simulink model "PD_trajectory"  (R2020b)
settings: Solver=VariableStepAuto  StartTime=0.0  StopTime=10  RelTol=1e-3
libraries: pid_lib x6
(part 1 of 3)
settings Model: Creator=Asus  LastModifiedBy=Asus

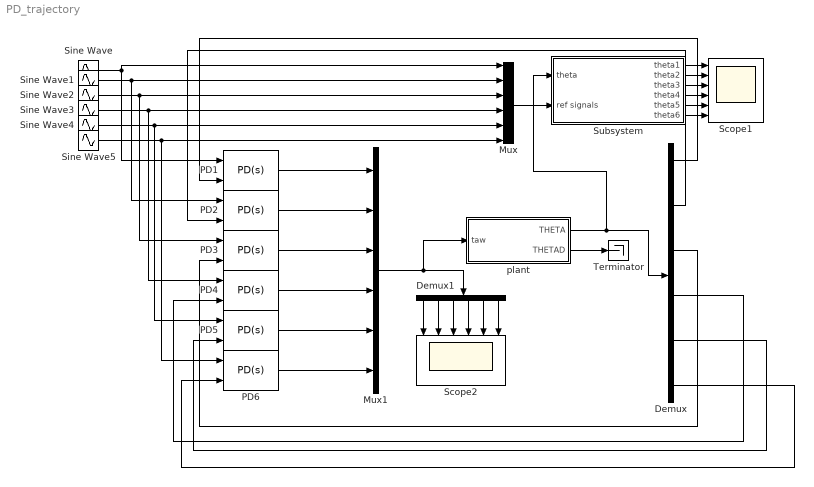
== system PD_trajectory ==
  Demux : Demux  Outputs=6
  Demux1 : Demux  Outputs=6
  Mux : Mux  Inputs=6
  Mux1 : Mux  Inputs=6
  PD1 : pid_lib/PID Controller (2DOF)  Controller=PD  Form=Parallel  TimeDomain=Continuous-time  UseExternalTs=off  SampleTime=-1  IntegratorMethod=Forward Euler  FilterMethod=Forward Euler  ControllerParametersSource=internal  P=343.666716329058  I=1  D=96720102.4595085  UseFilter=on  N=52762.3209030564  b=0.99828255964544  c=1.00028516180001  TunerSelectOption=Transfer Function Based (PID Tuner App)  InitialConditionSource=internal  InitialConditionForIntegrator=0  InitialConditionForFilter=0  DifferentiatorICPrevScaledInput=0  ExternalReset=none  TrackingMode=off  Kt=1  LimitOutput=off  SatLimitsSource=internal  UpperSaturationLimit=inf  LowerSaturationLimit=-inf  LinearizeAsGain=on  AntiWindupMode=none  Kb=1  POutMin=[]  POutMax=[]  IOutMin=[]  IOutMax=[]  DOutMin=[]  DOutMax=[]  NOutMin=[]  NOutMax=[]  bOutMin=[]  bOutMax=[]  cOutMin=[]  cOutMax=[]  SumOutMin=[]  SumOutMax=[]  SaturationOutMin=[]  SaturationOutMax=[]  PParamMin=[]  PParamMax=[]  IParamMin=[]  IParamMax=[]  DParamMin=[]  DParamMax=[]  NParamMin=[]  NParamMax=[]  bParamMin=[]  bParamMax=[]  cParamMin=[]  cParamMax=[]  KbParamMin=[]  KbParamMax=[]  KtParamMin=[]  KtParamMax=[]  KbOutMin=[]  KbOutMax=[]  KtOutMin=[]  KtOutMax=[]  IntegratorOutMin=[]  IntegratorOutMax=[]  FilterOutMin=[]  FilterOutMax=[]  SumI1OutMin=[]  SumI1OutMax=[]  SumI2OutMin=[]  SumI2OutMax=[]  SumI3OutMin=[]  SumI3OutMax=[]  SumI4OutMin=[]  SumI4OutMax=[]  SumDOutMin=[]  SumDOutMax=[]  Sum1OutMin=[]  Sum1OutMax=[]  Sum2OutMin=[]  Sum2OutMax=[]  Sum3OutMin=[]  Sum3OutMax=[]  DifferentiatorOutMin=[]  DifferentiatorOutMax=[]  FilterDiffOutCoefMin=[]  FilterDiffOutCoefMax=[]  ReciprocalOutMin=[]  ReciprocalOutMax=[]  SumDenOutMin=[]  SumDenOutMax=[]  SumNumOutMin=[]  SumNumOutMax=[]  DivideOutMin=[]  DivideOutMax=[]  UdiffTsProdOutMin=[]  UdiffTsProdOutMax=[]  NTsProdOutMin=[]  NTsProdOutMax=[]  UintegralTsProdOutMin=[]  UintegralTsProdOutMax=[]  UngainTsProdOutMin=[]  UngainTsProdOutMax=[]  IntegratorContinuousStateAttributes=''  IntegratorStateMustResolveToSignalObject=off  IntegratorRTWStateStorageClass=Auto  FilterContinuousStateAttributes=''  FilterStateMustResolveToSignalObject=off  FilterRTWStateStorageClass=Auto  ParallelPVariant=InternalParameters  IdealPVariant=Disabled  IVariant=Disabled  DVariant=InternalParameters  bVariant=InternalParameters  cVariant=InternalParameters  IntegratorVariant=Disabled  SatVariant=Disabled  AWVariant=Disabled  PCopyVariant=Disabled  TRVariant=Disabled  FdbkBlocksVariant=Forward  IdealPFdbkVariant=Disabled  SatFdbkVariant=Disabled  DerivativeFilterVariant=ContFilter  NVariant=InternalParameters  NCopyVariant=Disabled  FilterICVariant=InternalICsFilter  IntegratorICVariant=Disabled  ExternalResetVariant=Disabled  TRSumVariant=Passthrough  SumFdbkVariant=Disabled  SumVariant=Sum_PD  TsampFilterVariant=InternalTs  TsampNgainVariant=Passthrough  TsampIntegralVariant=Disabled_SignalSpec  ExternalSaturationOutDataTypeStr=Inherit: Same as second input
      settings: SourceProductBaseCode=SL
  PD2 : pid_lib/PID Controller (2DOF)  Controller=PD  Form=Parallel  TimeDomain=Continuous-time  UseExternalTs=off  SampleTime=-1  IntegratorMethod=Forward Euler  FilterMethod=Forward Euler  ControllerParametersSource=internal  P=119.449452109336  I=1  D=257028475.263143  UseFilter=on  N=212.729402533047  b=0.998165843121565  c=0.998149771769983  TunerSelectOption=Transfer Function Based (PID Tuner App)  InitialConditionSource=internal  InitialConditionForIntegrator=0  InitialConditionForFilter=0  DifferentiatorICPrevScaledInput=0  ExternalReset=none  TrackingMode=off  Kt=1  LimitOutput=off  SatLimitsSource=internal  UpperSaturationLimit=inf  LowerSaturationLimit=-inf  LinearizeAsGain=on  AntiWindupMode=none  Kb=1  POutMin=[]  POutMax=[]  IOutMin=[]  IOutMax=[]  DOutMin=[]  DOutMax=[]  NOutMin=[]  NOutMax=[]  bOutMin=[]  bOutMax=[]  cOutMin=[]  cOutMax=[]  SumOutMin=[]  SumOutMax=[]  SaturationOutMin=[]  SaturationOutMax=[]  PParamMin=[]  PParamMax=[]  IParamMin=[]  IParamMax=[]  DParamMin=[]  DParamMax=[]  NParamMin=[]  NParamMax=[]  bParamMin=[]  bParamMax=[]  cParamMin=[]  cParamMax=[]  KbParamMin=[]  KbParamMax=[]  KtParamMin=[]  KtParamMax=[]  KbOutMin=[]  KbOutMax=[]  KtOutMin=[]  KtOutMax=[]  IntegratorOutMin=[]  IntegratorOutMax=[]  FilterOutMin=[]  FilterOutMax=[]  SumI1OutMin=[]  SumI1OutMax=[]  SumI2OutMin=[]  SumI2OutMax=[]  SumI3OutMin=[]  SumI3OutMax=[]  SumI4OutMin=[]  SumI4OutMax=[]  SumDOutMin=[]  SumDOutMax=[]  Sum1OutMin=[]  Sum1OutMax=[]  Sum2OutMin=[]  Sum2OutMax=[]  Sum3OutMin=[]  Sum3OutMax=[]  DifferentiatorOutMin=[]  DifferentiatorOutMax=[]  FilterDiffOutCoefMin=[]  FilterDiffOutCoefMax=[]  ReciprocalOutMin=[]  ReciprocalOutMax=[]  SumDenOutMin=[]  SumDenOutMax=[]  SumNumOutMin=[]  SumNumOutMax=[]  DivideOutMin=[]  DivideOutMax=[]  UdiffTsProdOutMin=[]  UdiffTsProdOutMax=[]  NTsProdOutMin=[]  NTsProdOutMax=[]  UintegralTsProdOutMin=[]  UintegralTsProdOutMax=[]  UngainTsProdOutMin=[]  UngainTsProdOutMax=[]  IntegratorContinuousStateAttributes=''  IntegratorStateMustResolveToSignalObject=off  IntegratorRTWStateStorageClass=Auto  FilterContinuousStateAttributes=''  FilterStateMustResolveToSignalObject=off  FilterRTWStateStorageClass=Auto  ParallelPVariant=InternalParameters  IdealPVariant=Disabled  IVariant=Disabled  DVariant=InternalParameters  bVariant=InternalParameters  cVariant=InternalParameters  IntegratorVariant=Disabled  SatVariant=Disabled  AWVariant=Disabled  PCopyVariant=Disabled  TRVariant=Disabled  FdbkBlocksVariant=Forward  IdealPFdbkVariant=Disabled  SatFdbkVariant=Disabled  DerivativeFilterVariant=ContFilter  NVariant=InternalParameters  NCopyVariant=Disabled  FilterICVariant=InternalICsFilter  IntegratorICVariant=Disabled  ExternalResetVariant=Disabled  TRSumVariant=Passthrough  SumFdbkVariant=Disabled  SumVariant=Sum_PD  TsampFilterVariant=InternalTs  TsampNgainVariant=Passthrough  TsampIntegralVariant=Disabled_SignalSpec  ExternalSaturationOutDataTypeStr=Inherit: Same as second input
      settings: SourceProductBaseCode=SL
  PD3 : pid_lib/PID Controller (2DOF)  Controller=PD  Form=Parallel  TimeDomain=Continuous-time  UseExternalTs=off  SampleTime=-1  IntegratorMethod=Forward Euler  FilterMethod=Forward Euler  ControllerParametersSource=internal  P=499.181809831466  I=1  D=110528555.643449  UseFilter=on  N=798.367864997195  b=1.00179719301928  c=0.997974203873763  TunerSelectOption=Transfer Function Based (PID Tuner App)  InitialConditionSource=internal  InitialConditionForIntegrator=0  InitialConditionForFilter=0  DifferentiatorICPrevScaledInput=0  ExternalReset=none  TrackingMode=off  Kt=1  LimitOutput=off  SatLimitsSource=internal  UpperSaturationLimit=inf  LowerSaturationLimit=-inf  LinearizeAsGain=on  AntiWindupMode=none  Kb=1  POutMin=[]  POutMax=[]  IOutMin=[]  IOutMax=[]  DOutMin=[]  DOutMax=[]  NOutMin=[]  NOutMax=[]  bOutMin=[]  bOutMax=[]  cOutMin=[]  cOutMax=[]  SumOutMin=[]  SumOutMax=[]  SaturationOutMin=[]  SaturationOutMax=[]  PParamMin=[]  PParamMax=[]  IParamMin=[]  IParamMax=[]  DParamMin=[]  DParamMax=[]  NParamMin=[]  NParamMax=[]  bParamMin=[]  bParamMax=[]  cParamMin=[]  cParamMax=[]  KbParamMin=[]  KbParamMax=[]  KtParamMin=[]  KtParamMax=[]  KbOutMin=[]  KbOutMax=[]  KtOutMin=[]  KtOutMax=[]  IntegratorOutMin=[]  IntegratorOutMax=[]  FilterOutMin=[]  FilterOutMax=[]  SumI1OutMin=[]  SumI1OutMax=[]  SumI2OutMin=[]  SumI2OutMax=[]  SumI3OutMin=[]  SumI3OutMax=[]  SumI4OutMin=[]  SumI4OutMax=[]  SumDOutMin=[]  SumDOutMax=[]  Sum1OutMin=[]  Sum1OutMax=[]  Sum2OutMin=[]  Sum2OutMax=[]  Sum3OutMin=[]  Sum3OutMax=[]  DifferentiatorOutMin=[]  DifferentiatorOutMax=[]  FilterDiffOutCoefMin=[]  FilterDiffOutCoefMax=[]  ReciprocalOutMin=[]  ReciprocalOutMax=[]  SumDenOutMin=[]  SumDenOutMax=[]  SumNumOutMin=[]  SumNumOutMax=[]  DivideOutMin=[]  DivideOutMax=[]  UdiffTsProdOutMin=[]  UdiffTsProdOutMax=[]  NTsProdOutMin=[]  NTsProdOutMax=[]  UintegralTsProdOutMin=[]  UintegralTsProdOutMax=[]  UngainTsProdOutMin=[]  UngainTsProdOutMax=[]  IntegratorContinuousStateAttributes=''  IntegratorStateMustResolveToSignalObject=off  IntegratorRTWStateStorageClass=Auto  FilterContinuousStateAttributes=''  FilterStateMustResolveToSignalObject=off  FilterRTWStateStorageClass=Auto  ParallelPVariant=InternalParameters  IdealPVariant=Disabled  IVariant=Disabled  DVariant=InternalParameters  bVariant=InternalParameters  cVariant=InternalParameters  IntegratorVariant=Disabled  SatVariant=Disabled  AWVariant=Disabled  PCopyVariant=Disabled  TRVariant=Disabled  FdbkBlocksVariant=Forward  IdealPFdbkVariant=Disabled  SatFdbkVariant=Disabled  DerivativeFilterVariant=ContFilter  NVariant=InternalParameters  NCopyVariant=Disabled  FilterICVariant=InternalICsFilter  IntegratorICVariant=Disabled  ExternalResetVariant=Disabled  TRSumVariant=Passthrough  SumFdbkVariant=Disabled  SumVariant=Sum_PD  TsampFilterVariant=InternalTs  TsampNgainVariant=Passthrough  TsampIntegralVariant=Disabled_SignalSpec  ExternalSaturationOutDataTypeStr=Inherit: Same as second input
      settings: SourceProductBaseCode=SL
  PD4 : pid_lib/PID Controller (2DOF)  Controller=PD  Form=Parallel  TimeDomain=Continuous-time  UseExternalTs=off  SampleTime=-1  IntegratorMethod=Forward Euler  FilterMethod=Forward Euler  ControllerParametersSource=internal  P=35.1765838870725  I=1  D=43623360.6425588  UseFilter=on  N=2375.55389046885  b=0.998970930122497  c=0.998724654187734  TunerSelectOption=Transfer Function Based (PID Tuner App)  InitialConditionSource=internal  InitialConditionForIntegrator=0  InitialConditionForFilter=0  DifferentiatorICPrevScaledInput=0  ExternalReset=none  TrackingMode=off  Kt=1  LimitOutput=off  SatLimitsSource=internal  UpperSaturationLimit=inf  LowerSaturationLimit=-inf  LinearizeAsGain=on  AntiWindupMode=none  Kb=1  POutMin=[]  POutMax=[]  IOutMin=[]  IOutMax=[]  DOutMin=[]  DOutMax=[]  NOutMin=[]  NOutMax=[]  bOutMin=[]  bOutMax=[]  cOutMin=[]  cOutMax=[]  SumOutMin=[]  SumOutMax=[]  SaturationOutMin=[]  SaturationOutMax=[]  PParamMin=[]  PParamMax=[]  IParamMin=[]  IParamMax=[]  DParamMin=[]  DParamMax=[]  NParamMin=[]  NParamMax=[]  bParamMin=[]  bParamMax=[]  cParamMin=[]  cParamMax=[]  KbParamMin=[]  KbParamMax=[]  KtParamMin=[]  KtParamMax=[]  KbOutMin=[]  KbOutMax=[]  KtOutMin=[]  KtOutMax=[]  IntegratorOutMin=[]  IntegratorOutMax=[]  FilterOutMin=[]  FilterOutMax=[]  SumI1OutMin=[]  SumI1OutMax=[]  SumI2OutMin=[]  SumI2OutMax=[]  SumI3OutMin=[]  SumI3OutMax=[]  SumI4OutMin=[]  SumI4OutMax=[]  SumDOutMin=[]  SumDOutMax=[]  Sum1OutMin=[]  Sum1OutMax=[]  Sum2OutMin=[]  Sum2OutMax=[]  Sum3OutMin=[]  Sum3OutMax=[]  DifferentiatorOutMin=[]  DifferentiatorOutMax=[]  FilterDiffOutCoefMin=[]  FilterDiffOutCoefMax=[]  ReciprocalOutMin=[]  ReciprocalOutMax=[]  SumDenOutMin=[]  SumDenOutMax=[]  SumNumOutMin=[]  SumNumOutMax=[]  DivideOutMin=[]  DivideOutMax=[]  UdiffTsProdOutMin=[]  UdiffTsProdOutMax=[]  NTsProdOutMin=[]  NTsProdOutMax=[]  UintegralTsProdOutMin=[]  UintegralTsProdOutMax=[]  UngainTsProdOutMin=[]  UngainTsProdOutMax=[]  IntegratorContinuousStateAttributes=''  IntegratorStateMustResolveToSignalObject=off  IntegratorRTWStateStorageClass=Auto  FilterContinuousStateAttributes=''  FilterStateMustResolveToSignalObject=off  FilterRTWStateStorageClass=Auto  ParallelPVariant=InternalParameters  IdealPVariant=Disabled  IVariant=Disabled  DVariant=InternalParameters  bVariant=InternalParameters  cVariant=InternalParameters  IntegratorVariant=Disabled  SatVariant=Disabled  AWVariant=Disabled  PCopyVariant=Disabled  TRVariant=Disabled  FdbkBlocksVariant=Forward  IdealPFdbkVariant=Disabled  SatFdbkVariant=Disabled  DerivativeFilterVariant=ContFilter  NVariant=InternalParameters  NCopyVariant=Disabled  FilterICVariant=InternalICsFilter  IntegratorICVariant=Disabled  ExternalResetVariant=Disabled  TRSumVariant=Passthrough  SumFdbkVariant=Disabled  SumVariant=Sum_PD  TsampFilterVariant=InternalTs  TsampNgainVariant=Passthrough  TsampIntegralVariant=Disabled_SignalSpec  ExternalSaturationOutDataTypeStr=Inherit: Same as second input
      settings: SourceProductBaseCode=SL
  PD5 : pid_lib/PID Controller (2DOF)  Controller=PD  Form=Parallel  TimeDomain=Continuous-time  UseExternalTs=off  SampleTime=-1  IntegratorMethod=Forward Euler  FilterMethod=Forward Euler  ControllerParametersSource=internal  P=202884107.344588  I=1  D=8509.35091124406  UseFilter=on  N=100856.735690592  b=0.998513041388824  c=0.422810076890989  TunerSelectOption=Transfer Function Based (PID Tuner App)  InitialConditionSource=internal  InitialConditionForIntegrator=0  InitialConditionForFilter=0  DifferentiatorICPrevScaledInput=0  ExternalReset=none  TrackingMode=off  Kt=1  LimitOutput=off  SatLimitsSource=internal  UpperSaturationLimit=inf  LowerSaturationLimit=-inf  LinearizeAsGain=on  AntiWindupMode=none  Kb=1  POutMin=[]  POutMax=[]  IOutMin=[]  IOutMax=[]  DOutMin=[]  DOutMax=[]  NOutMin=[]  NOutMax=[]  bOutMin=[]  bOutMax=[]  cOutMin=[]  cOutMax=[]  SumOutMin=[]  SumOutMax=[]  SaturationOutMin=[]  SaturationOutMax=[]  PParamMin=[]  PParamMax=[]  IParamMin=[]  IParamMax=[]  DParamMin=[]  DParamMax=[]  NParamMin=[]  NParamMax=[]  bParamMin=[]  bParamMax=[]  cParamMin=[]  cParamMax=[]  KbParamMin=[]  KbParamMax=[]  KtParamMin=[]  KtParamMax=[]  KbOutMin=[]  KbOutMax=[]  KtOutMin=[]  KtOutMax=[]  IntegratorOutMin=[]  IntegratorOutMax=[]  FilterOutMin=[]  FilterOutMax=[]  SumI1OutMin=[]  SumI1OutMax=[]  SumI2OutMin=[]  SumI2OutMax=[]  SumI3OutMin=[]  SumI3OutMax=[]  SumI4OutMin=[]  SumI4OutMax=[]  SumDOutMin=[]  SumDOutMax=[]  Sum1OutMin=[]  Sum1OutMax=[]  Sum2OutMin=[]  Sum2OutMax=[]  Sum3OutMin=[]  Sum3OutMax=[]  DifferentiatorOutMin=[]  DifferentiatorOutMax=[]  FilterDiffOutCoefMin=[]  FilterDiffOutCoefMax=[]  ReciprocalOutMin=[]  ReciprocalOutMax=[]  SumDenOutMin=[]  SumDenOutMax=[]  SumNumOutMin=[]  SumNumOutMax=[]  DivideOutMin=[]  DivideOutMax=[]  UdiffTsProdOutMin=[]  UdiffTsProdOutMax=[]  NTsProdOutMin=[]  NTsProdOutMax=[]  UintegralTsProdOutMin=[]  UintegralTsProdOutMax=[]  UngainTsProdOutMin=[]  UngainTsProdOutMax=[]  IntegratorContinuousStateAttributes=''  IntegratorStateMustResolveToSignalObject=off  IntegratorRTWStateStorageClass=Auto  FilterContinuousStateAttributes=''  FilterStateMustResolveToSignalObject=off  FilterRTWStateStorageClass=Auto  ParallelPVariant=InternalParameters  IdealPVariant=Disabled  IVariant=Disabled  DVariant=InternalParameters  bVariant=InternalParameters  cVariant=InternalParameters  IntegratorVariant=Disabled  SatVariant=Disabled  AWVariant=Disabled  PCopyVariant=Disabled  TRVariant=Disabled  FdbkBlocksVariant=Forward  IdealPFdbkVariant=Disabled  SatFdbkVariant=Disabled  DerivativeFilterVariant=ContFilter  NVariant=InternalParameters  NCopyVariant=Disabled  FilterICVariant=InternalICsFilter  IntegratorICVariant=Disabled  ExternalResetVariant=Disabled  TRSumVariant=Passthrough  SumFdbkVariant=Disabled  SumVariant=Sum_PD  TsampFilterVariant=InternalTs  TsampNgainVariant=Passthrough  TsampIntegralVariant=Disabled_SignalSpec  ExternalSaturationOutDataTypeStr=Inherit: Same as second input
      settings: SourceProductBaseCode=SL
  PD6 : pid_lib/PID Controller (2DOF)  Controller=PD  Form=Parallel  TimeDomain=Continuous-time  UseExternalTs=off  SampleTime=-1  IntegratorMethod=Forward Euler  FilterMethod=Forward Euler  ControllerParametersSource=internal  P=3.97815719463879  I=1  D=2.18754227101202  UseFilter=on  N=576133.716100811  b=1.00180101217612  c=1.06274606142442  TunerSelectOption=Transfer Function Based (PID Tuner App)  InitialConditionSource=internal  InitialConditionForIntegrator=0  InitialConditionForFilter=0  DifferentiatorICPrevScaledInput=0  ExternalReset=none  TrackingMode=off  Kt=1  LimitOutput=off  SatLimitsSource=internal  UpperSaturationLimit=inf  LowerSaturationLimit=-inf  LinearizeAsGain=on  AntiWindupMode=none  Kb=1  POutMin=[]  POutMax=[]  IOutMin=[]  IOutMax=[]  DOutMin=[]  DOutMax=[]  NOutMin=[]  NOutMax=[]  bOutMin=[]  bOutMax=[]  cOutMin=[]  cOutMax=[]  SumOutMin=[]  SumOutMax=[]  SaturationOutMin=[]  SaturationOutMax=[]  PParamMin=[]  PParamMax=[]  IParamMin=[]  IParamMax=[]  DParamMin=[]  DParamMax=[]  NParamMin=[]  NParamMax=[]  bParamMin=[]  bParamMax=[]  cParamMin=[]  cParamMax=[]  KbParamMin=[]  KbParamMax=[]  KtParamMin=[]  KtParamMax=[]  KbOutMin=[]  KbOutMax=[]  KtOutMin=[]  KtOutMax=[]  IntegratorOutMin=[]  IntegratorOutMax=[]  FilterOutMin=[]  FilterOutMax=[]  SumI1OutMin=[]  SumI1OutMax=[]  SumI2OutMin=[]  SumI2OutMax=[]  SumI3OutMin=[]  SumI3OutMax=[]  SumI4OutMin=[]  SumI4OutMax=[]  SumDOutMin=[]  SumDOutMax=[]  Sum1OutMin=[]  Sum1OutMax=[]  Sum2OutMin=[]  Sum2OutMax=[]  Sum3OutMin=[]  Sum3OutMax=[]  DifferentiatorOutMin=[]  DifferentiatorOutMax=[]  FilterDiffOutCoefMin=[]  FilterDiffOutCoefMax=[]  ReciprocalOutMin=[]  ReciprocalOutMax=[]  SumDenOutMin=[]  SumDenOutMax=[]  SumNumOutMin=[]  SumNumOutMax=[]  DivideOutMin=[]  DivideOutMax=[]  UdiffTsProdOutMin=[]  UdiffTsProdOutMax=[]  NTsProdOutMin=[]  NTsProdOutMax=[]  UintegralTsProdOutMin=[]  UintegralTsProdOutMax=[]  UngainTsProdOutMin=[]  UngainTsProdOutMax=[]  IntegratorContinuousStateAttributes=''  IntegratorStateMustResolveToSignalObject=off  IntegratorRTWStateStorageClass=Auto  FilterContinuousStateAttributes=''  FilterStateMustResolveToSignalObject=off  FilterRTWStateStorageClass=Auto  ParallelPVariant=InternalParameters  IdealPVariant=Disabled  IVariant=Disabled  DVariant=InternalParameters  bVariant=InternalParameters  cVariant=InternalParameters  IntegratorVariant=Disabled  SatVariant=Disabled  AWVariant=Disabled  PCopyVariant=Disabled  TRVariant=Disabled  FdbkBlocksVariant=Forward  IdealPFdbkVariant=Disabled  SatFdbkVariant=Disabled  DerivativeFilterVariant=ContFilter  NVariant=InternalParameters  NCopyVariant=Disabled  FilterICVariant=InternalICsFilter  IntegratorICVariant=Disabled  ExternalResetVariant=Disabled  TRSumVariant=Passthrough  SumFdbkVariant=Disabled  SumVariant=Sum_PD  TsampFilterVariant=InternalTs  TsampNgainVariant=Passthrough  TsampIntegralVariant=Disabled_SignalSpec  ExternalSaturationOutDataTypeStr=Inherit: Same as second input
      settings: SourceProductBaseCode=SL
  Scope1 : Scope  NumInputPorts=6
  Scope2 : Scope  NumInputPorts=6
  Sine Wave{,1..5} (6 alike) : Sin  SampleTime=0
  Subsystem : Subsystem
  Terminator : Terminator
  plant : Subsystem
  wires:
  PD5/1 -> Mux1/5
  Demux/6 -> PD6/2
  PD1/1 -> Mux1/1
  PD4/1 -> Mux1/4
  Demux/3 -> PD3/2
  PD3/1 -> Mux1/3
  PD6/1 -> Mux1/6
  Demux/2 -> PD2/2
  Mux1/1 -> Demux1/1, plant/1(taw)
  Demux/1 -> PD1/2
  Sine Wave5/1 -> PD6/1, Mux/6
  Demux/5 -> PD5/2
  Sine Wave/1 -> Mux/1, PD1/1
  Sine Wave2/1 -> PD3/1, Mux/3
  Demux/4 -> PD4/2
  plant/1(THETA) -> Subsystem/1(theta), Demux/1
  plant/2(THETAD) -> Terminator/1
  Sine Wave3/1 -> PD4/1, Mux/4
  Sine Wave4/1 -> PD5/1, Mux/5
  Sine Wave1/1 -> PD2/1, Mux/2
  PD2/1 -> Mux1/2
  Subsystem/4(theta4) -> Scope1/4
  Subsystem/6(theta6) -> Scope1/6
  Subsystem/5(theta5) -> Scope1/5
  Subsystem/3(theta3) -> Scope1/3
  Mux/1 -> Subsystem/2(ref signals)
  Subsystem/2(theta2) -> Scope1/2
  Subsystem/1(theta1) -> Scope1/1
  Demux1/2 -> Scope2/2
  Demux1/5 -> Scope2/5
  Demux1/1 -> Scope2/1
  Demux1/6 -> Scope2/6
  Demux1/4 -> Scope2/4
  Demux1/3 -> Scope2/3

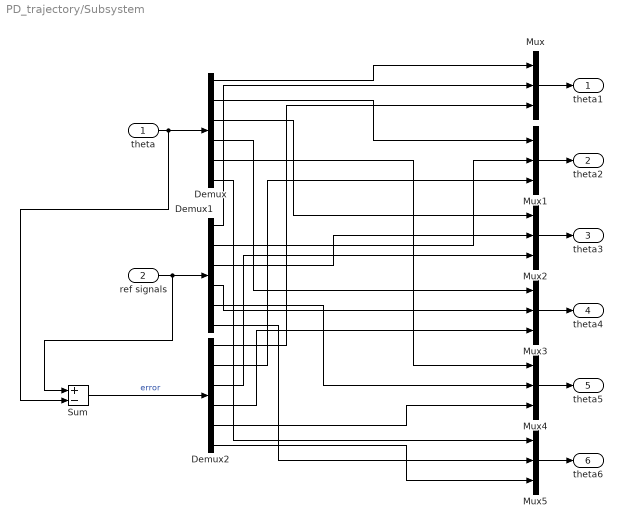
== system PD_trajectory/Subsystem ==
  theta : Inport
  ref signals : Inport  Port=2
  Demux : Demux  Outputs=6
  Demux1 : Demux  Outputs=6
  Demux2 : Demux  Outputs=6
  Mux{,1..5} (6 alike) : Mux  Inputs=3
  Sum : Sum  Inputs=+-
  theta1 : Outport
  theta2 : Outport  Port=2
  theta3 : Outport  Port=3
  theta4 : Outport  Port=4
  theta5 : Outport  Port=5
  theta6 : Outport  Port=6
  wires:
  Mux/1 -> theta1/1
  Mux1/1 -> theta2/1
  Mux2/1 -> theta3/1
  Mux5/1 -> theta6/1
  Mux4/1 -> theta5/1
  Mux3/1 -> theta4/1
  theta/1 -> Sum/2, Demux/1
  ref signals/1 -> Sum/1, Demux1/1
  Sum/1 -> Demux2/1  "error"
  Demux/1 -> Mux/1
  Demux/2 -> Mux1/1
  Demux/3 -> Mux2/1
  Demux/4 -> Mux3/1
  Demux/5 -> Mux4/1
  Demux/6 -> Mux5/1
  Demux1/1 -> Mux/2
  Demux1/2 -> Mux1/2
  Demux1/3 -> Mux2/2
  Demux1/4 -> Mux3/2
  Demux1/5 -> Mux4/2
  Demux1/6 -> Mux5/2
  Demux2/6 -> Mux5/3
  Demux2/5 -> Mux4/3
  Demux2/4 -> Mux3/3
  Demux2/3 -> Mux2/3
  Demux2/2 -> Mux1/3
  Demux2/1 -> Mux/3

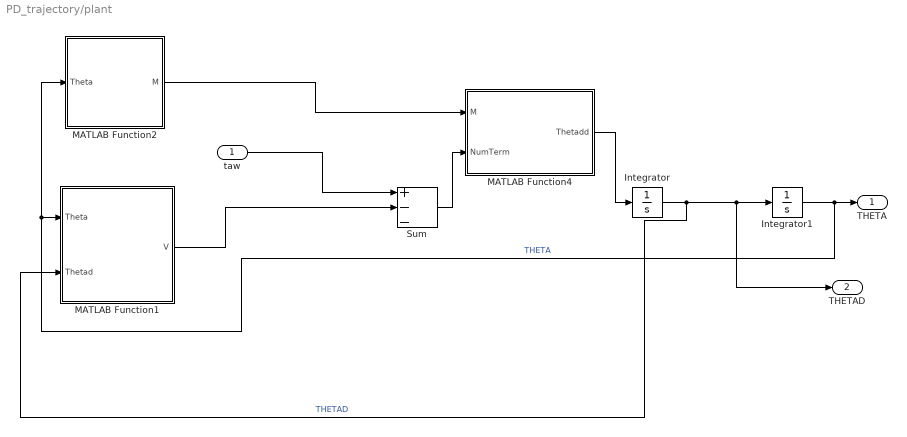
== system PD_trajectory/plant ==
  taw : Inport
  Integrator : Integrator  InitialCondition=[0,0,0,0,0,0]
  Integrator1 : Integrator  InitialCondition=[0,0,0,0,0,0]
  MATLAB Function1 : MATLAB Function  TreatAsAtomicUnit=on
  MATLAB Function2 : MATLAB Function  TreatAsAtomicUnit=on
  MATLAB Function4 : MATLAB Function  TreatAsAtomicUnit=on
  Sum : Sum  Inputs=+--
  THETA : Outport
  THETAD : Outport  Port=2
  wires:
  Integrator/1 -> MATLAB Function1/2(Thetad), THETAD/1, Integrator1/1  "THETAD"
  MATLAB Function4/1(Thetadd) -> Integrator/1
  MATLAB Function1/1(V) -> Sum/2
  MATLAB Function2/1(M) -> MATLAB Function4/1(M)
  Sum/1 -> MATLAB Function4/2(NumTerm)
  Integrator1/1 -> MATLAB Function1/1(Theta), MATLAB Function2/1(Theta), THETA/1  "THETA"
  taw/1 -> Sum/1

== matlab function PD_trajectory/plant/MATLAB Function2 ==
  data: Theta input; M output
function M = NumM(Theta)
t1=Theta(1);
t2=Theta(2);
t3=Theta(3);
t4=Theta(4);
t5=Theta(5);
t6=Theta(6);

L1=0.1025;
L2=0.408;
L3=0.376;
L4=0.1025; 
L5=0.1025;


M=zeros(6);
M(1)=(999498*cos(t3 + t4))/5 - (9799*L4)/40 - (33481296*cos(2*t2 + t3))/25 -...
    (30203396714246934648101547*cos(2*t2))/28823037615171174400 - (401759*cos(2*t2 + 2*t3 + 2*t4))/16 -...
    (15427656*cos(2*t2 + 2*t3))/25 - (999498*cos(2*t2 + t3 + t4))/5 - (219461*L1)/100 + (33481296*cos(t3))/25 +...
    (921106*cos(t4))/5 - (921106*cos(2*t2 + 2*t3 + t4))/5 - (239*L3^2*cos(2*t2 + 2*t3 + 2*t4 - 2*t5))/3200 -...
    (239*L3^2*cos(2*t2 + 2*t3 + 2*t4 + 2*t5))/3200 + (24378*L4*cos(2*t2 + t3 + t4))/25 +...
    (12189*L3*cos(t3 + t4 - t5))/50 - (757*L2^2*cos(2*t2))/800 + (239*L3^2*cos(2*t5))/1600 +...
    (239*L3^2*cos(2*t2 + 2*t3 + 2*t4))/1600 - (239*L4^2*cos(2*t2 + 2*t3 + 2*t4))/200 - (24378*L4*cos(t3 + t4))/25 -...
    (11233*L3*cos(t4 + t5))/50 - (11233*L3*cos(2*t2 + 2*t3 + t4 - t5))/50 + (9799*L3*cos(2*t2 + 2*t3 + 2*t4 + t5))/160 +...
    (67159*L3*cos(t5))/200 - (22466*L4*cos(t4))/25 + (22466*L4*cos(2*t2 + 2*t3 + t4))/25 +...
    (12189*L3*cos(2*t2 + t3 + t4 + t5))/50 + (781*L1^2)/100 + (757*L2^2)/800 + (717*L3^2)/1600 +...
    (239*L4^2)/200 + (11233*L3*cos(t4 - t5))/50 - (9799*L3*cos(2*t2 + 2*t3 + 2*t4 - t5))/160 -...
    (12189*L3*cos(t3 + t4 + t5))/50 + (9799*L4*cos(2*t2 + 2*t3 + 2*t4))/40 -...
    (12189*L3*cos(2*t2 + t3 + t4 - t5))/50 + (11233*L3*cos(2*t2 + 2*t3 + t4 + t5))/50 +...
    (239*L3*L4*cos(2*t2 + 2*t3 + 2*t4 - t5))/400 - (239*L3*L4*cos(2*t2 + 2*t3 + 2*t4 + t5))/400 +...
    60184539611691967063155889/28823037615171174400;
M(7)=(61463515545781917*cos(t1 + 2*t2))/2305843009213693952 - (61463515545781917*cos(t1 - 2*t2))/2305843009213693952 -...
    (2753519*cos(t2 + t3 + t4))/40 - (11529711*cos(t2 + t3))/25 - (18042729*cos(t2))/25 - (757*L2^2*cos(t1 - 2*t2))/1600 +...
    (757*L2^2*cos(t1 + 2*t2))/1600 - (11233*L3*cos(t2 + t3 - t5))/50 + (4541*L3*cos(t2 + t3 + t4 + t5))/200 -...
    (212717*L2*cos(t1 + t2))/800 + (7426*L1*cos(t2 + t3))/5 - (12189*L3*cos(t2 + t5))/50 + (79662*L1*cos(t2))/25 -...
    (58077*L3*cos(t2 + t3 + t4 - t5))/400 - (212717*L2*cos(t1 - t2))/800 - (12189*L3*cos(t2 - t5))/50 -...
    (11233*L3*cos(t2 + t3 + t5))/50 + (67159*L4*cos(t2 + t3 + t4))/200 - (239*L3^2*cos(t2 + t3 + t4 - 2*t5))/1600 +...
    (239*L3^2*cos(t2 + t3 + t4 + 2*t5))/1600 + (239*L3*L4*cos(t2 + t3 + t4 + t5))/400 +...
    (239*L3*L4*cos(t2 + t3 + t4 - t5))/400;
M(13)=(1690603261718859*cos(t1 - 2*t2))/2305843009213693952 - (1690603261718859*cos(t1 + 2*t2))/2305843009213693952 -...
    (2753519*cos(t2 + t3 + t4))/40 - (11529711*cos(t2 + t3))/25 - (11233*L3*cos(t2 + t3 - t5))/50 +...
    (4541*L3*cos(t2 + t3 + t4 + t5))/200 + (7426*L1*cos(t2 + t3))/5 - (58077*L3*cos(t2 + t3 + t4 - t5))/400 -...
    (11233*L3*cos(t2 + t3 + t5))/50 + (67159*L4*cos(t2 + t3 + t4))/200 - (239*L3^2*cos(t2 + t3 + t4 - 2*t5))/1600 +...
    (239*L3^2*cos(t2 + t3 + t4 + 2*t5))/1600 + (239*L3*L4*cos(t2 + t3 + t4 + t5))/400 +...
    (239*L3*L4*cos(t2 + t3 + t4 - t5))/400;
M(19)=(1690603261718859*cos(t1 - 2*t2))/2305843009213693952 - (1690603261718859*cos(t1 + 2*t2))/2305843009213693952 -...
    (2753519*cos(t2 + t3 + t4))/40 + (4541*L3*cos(t2 + t3 + t4 + t5))/200 - (58077*L3*cos(t2 + t3 + t4 - t5))/400 +...
    (67159*L4*cos(t2 + t3 + t4))/200 - (239*L3^2*cos(t2 + t3 + t4 - 2*t5))/1600 + (239*L3^2*cos(t2 + t3 + t4 + 2*t5))/1600 +...
    (239*L3*L4*cos(t2 + t3 + t4 + t5))/400 + (239*L3*L4*cos(t2 + t3 + t4 - t5))/400;
M(25)=(1690603261718859*cos(t2 + t3 + t4))/1152921504606846976 - (1690603261718859*cos(t1 + t2 - t3 - t4))/4611686018427387904 +...
    (1690603261718859*cos(3*t2 - t1 + t3 + t4))/4611686018427387904 - (1690603261718859*cos(t3 - t2 + t4))/2305843009213693952 -...
    (1690603261718859*cos(3*t2 + t3 + t4))/2305843009213693952 - (1690603261718859*cos(t1 - t2 + t3 + t4))/4611686018427387904 +...
    (1690603261718859*cos(t1 + 3*t2 + t3 + t4))/4611686018427387904 - (11233*L3*cos(t2 + t3 - t5))/50 + (239*L3^2*cos(t2 + t3 + t4))/400 +...
    (58077*L3*cos(t2 + t3 + t4 + t5))/400 + (12189*L3*cos(t2 + t5))/50 + (4541*L3*cos(t2 + t3 + t4 - t5))/200 - (12189*L3*cos(t2 - t5))/50 +...
    (11233*L3*cos(t2 + t3 + t5))/50 - (239*L3*L4*cos(t2 + t3 + t4 + t5))/400 + (239*L3*L4*cos(t2 + t3 + t4 - t5))/400;
M(31)=0;
M(2)=(61463515545781917*cos(t1 + 2*t2))/2305843009213693952 - (61463515545781917*cos(t1 - 2*t2))/2305843009213693952 -...
    (2753519*cos(t2 + t3 + t4))/40 - (11529711*cos(t2 + t3))/25 - (18042729*cos(t2))/25 - (757*L2^2*cos(t1 - 2*t2))/1600 +...
    (757*L2^2*cos(t1 + 2*t2))/1600 - (11233*L3*cos(t2 + t3 - t5))/50 + (4541*L3*cos(t2 + t3 + t4 + t5))/200 -...
    (212717*L2*cos(t1 + t2))/800 + (7426*L1*cos(t2 + t3))/5 - (12189*L3*cos(t2 + t5))/50 + (79662*L1*cos(t2))/25 -...
    (58077*L3*cos(t2 + t3 + t4 - t5))/400 - (212717*L2*cos(t1 - t2))/800 - (12189*L3*cos(t2 - t5))/50 -...
    (11233*L3*cos(t2 + t3 + t5))/50 + (67159*L4*cos(t2 + t3 + t4))/200 - (239*L3^2*cos(t2 + t3 + t4 - 2*t5))/1600 +...
    (239*L3^2*cos(t2 + t3 + t4 + 2*t5))/1600 + (239*L3*L4*cos(t2 + t3 + t4 + t5))/400 + (239*L3*L4*cos(t2 + t3 + t4 - t5))/400;
M(8)=(66962592*cos(t3))/25 - (9799*L4)/20 + (1842212*cos(t4))/5 + (1998996*cos(t3)*cos(t4))/5 - (1998996*sin(t3)*sin(t4))/5 -...
    (17228543827841635967893663*cos(t1)^2)/115292150460684697600 - (61463515545781917*cos(t2)^2)/576460752303423488 +...
    (1690603261718859*cos(t3)^2)/576460752303423488 + (757*L2^2*cos(t1)^2)/400 + (757*L2^2*cos(t2)^2)/400 -...
    (239*L3^2*cos(t5)^2)/400 - (44932*L4*cos(t4))/25 + (239*L3^2)/400 + (239*L4^2)/100 + ...
    (61463515545781917*cos(t1)^2*cos(t2)^2)/576460752303423488 - (1690603261718859*cos(t1)^2*cos(t3)^2)/288230376151711744 -...
    (48756*L4*cos(t3)*cos(t4))/25 - (757*L2^2*cos(t1)^2*cos(t2)^2)/400 + (48756*L4*sin(t3)*sin(t4))/25 + (22466*L3*sin(t4)*sin(t5))/25 -...
    (212717*L2*cos(t1)*sin(t1)*sin(t2))/200 + (24378*L3*cos(t3)*sin(t4)*sin(t5))/25 + (24378*L3*cos(t4)*sin(t3)*sin(t5))/25 -...
    (1690603261718859*cos(t1)*cos(t3)*sin(t1)*sin(t3))/288230376151711744 + 406940712223380376880235337/115292150460684697600;
M(14)=(33481296*cos(t3))/25 - (9799*L4)/20 + (1842212*cos(t4))/5 + (999498*cos(t3)*cos(t4))/5 - (999498*sin(t3)*sin(t4))/5 +...
    (22503512638915017*cos(t1)^2)/4611686018427387904 + (1690603261718859*cos(t2)^2)/576460752303423488 +...
    (1690603261718859*cos(t3)^2)/576460752303423488 - (239*L3^2*cos(t5)^2)/400 - (44932*L4*cos(t4))/25 +...
    (239*L3^2)/400 + (239*L4^2)/100 - (1690603261718859*cos(t1)^2*cos(t2)^2)/576460752303423488 -...
    (1690603261718859*cos(t1)^2*cos(t3)^2)/288230376151711744 - (24378*L4*cos(t3)*cos(t4))/25 +...
    (24378*L4*sin(t3)*sin(t4))/25 + (22466*L3*sin(t4)*sin(t5))/25 + (12189*L3*cos(t3)*sin(t4)*sin(t5))/25 +...
    (12189*L3*cos(t4)*sin(t3)*sin(t5))/25 - (1690603261718859*cos(t1)*cos(t3)*sin(t1)*sin(t3))/288230376151711744 +...
    148084969195448577098115273/115292150460684697600;
M(20)=(24162136260015883*cos(2*t1))/9223372036854775808 - (9799*L4)/20 + (1690603261718859*cos(2*t2))/2305843009213693952 +...
    (921106*cos(t4))/5 + (999498*cos(t3)*cos(t4))/5 - (999498*sin(t3)*sin(t4))/5 - (239*L3^2*cos(t5)^2)/400 -...
    (22466*L4*cos(t4))/25 + (239*L3^2)/400 + (239*L4^2)/100 - (1690603261718859*cos(2*t1)*cos(2*t2))/2305843009213693952 -...
    (1690603261718859*cos(2*t1)*cos(t3)^2)/576460752303423488 - (24378*L4*cos(t3)*cos(t4))/25 -...
    (1690603261718859*sin(2*t1)*cos(t3)*sin(t3))/576460752303423488 + (24378*L4*sin(t3)*sin(t4))/25 +...
    (11233*L3*sin(t4)*sin(t5))/25 + (12189*L3*cos(t3)*sin(t4)*sin(t5))/25 + (12189*L3*cos(t4)*sin(t3)*sin(t5))/25 +...
    463196680911590935827689/9223372036854775808;
M(26)=(1690603261718859*cos(2*t1 + t2 - t3 + t4))/2305843009213693952 - (1690603261718859*cos(t1 + t2 - t3 - t4))/4611686018427387904 +...
    (1690603261718859*cos(2*t1 - t2 + t3 + t4))/9223372036854775808 + (1690603261718859*cos(3*t2 - t1 + t3 + t4))/4611686018427387904 -...
    (1690603261718859*cos(t2 - 2*t1 + 3*t3 + t4))/2305843009213693952 - (1690603261718859*cos(3*t2 - 2*t1 + t3 + t4))/9223372036854775808 +...
    (1690603261718859*cos(2*t1 + 3*t2 + t3 + t4))/9223372036854775808 - (1690603261718859*cos(2*t1 + t2 - t3 - t4))/9223372036854775808 +...
    (1690603261718859*cos(t1 - t2 + t3 + t4))/4611686018427387904 + (10637310166265011*cos(t2 - 2*t1 + t3 + t4))/18446744073709551616 -...
    (10637310166265011*cos(2*t1 + t2 + t3 + t4))/18446744073709551616 - (1690603261718859*cos(t1 + 3*t2 + t3 + t4))/4611686018427387904 -...
    (12189*L3*cos(t3 + t4 - t5))/50 - (11233*L3*cos(t4 + t5))/50 - (9799*L3*cos(t5))/80 - (11233*L3*cos(t4 - t5))/50 -...
    (12189*L3*cos(t3 + t4 + t5))/50 + (239*L3*L4*cos(t5))/200;
M(32)=(3874897119389575*cos(t5))/4611686018427387904 + (3874897119389575*cos(t1)^2*cos(t5))/4611686018427387904 -...
    (3874897119389575*cos(t1)*cos(t2)*cos(t3)*cos(t4)*sin(t1)*sin(t5))/4611686018427387904 +...
    (3874897119389575*cos(t1)*cos(t2)*sin(t1)*sin(t3)*sin(t4)*sin(t5))/4611686018427387904 +...
    (3874897119389575*cos(t1)*cos(t3)*sin(t1)*sin(t2)*sin(t4)*sin(t5))/4611686018427387904 +...
    (3874897119389575*cos(t1)*cos(t4)*sin(t1)*sin(t2)*sin(t3)*sin(t5))/4611686018427387904;
M(3)=(1690603261718859*cos(t1 - 2*t2))/2305843009213693952 - (1690603261718859*cos(t1 + 2*t2))/2305843009213693952 -...
    (2753519*cos(t2 + t3 + t4))/40 - (11529711*cos(t2 + t3))/25 - (11233*L3*cos(t2 + t3 - t5))/50 +...
    (4541*L3*cos(t2 + t3 + t4 + t5))/200 + (7426*L1*cos(t2 + t3))/5 - (58077*L3*cos(t2 + t3 + t4 - t5))/400 -...
    (11233*L3*cos(t2 + t3 + t5))/50 + (67159*L4*cos(t2 + t3 + t4))/200 - (239*L3^2*cos(t2 + t3 + t4 - 2*t5))/1600 +...
    (239*L3^2*cos(t2 + t3 + t4 + 2*t5))/1600 + (239*L3*L4*cos(t2 + t3 + t4 + t5))/400 +...
    (239*L3*L4*cos(t2 + t3 + t4 - t5))/400;
M(9)=(33481296*cos(t3))/25 - (9799*L4)/20 + (1842212*cos(t4))/5 + (999498*cos(t3)*cos(t4))/5 - (999498*sin(t3)*sin(t4))/5 +...
    (22503512638915017*cos(t1)^2)/4611686018427387904 + (1690603261718859*cos(t2)^2)/576460752303423488 + ...
    (1690603261718859*cos(t3)^2)/576460752303423488 - (239*L3^2*cos(t5)^2)/400 - (44932*L4*cos(t4))/25 + ...
    (239*L3^2)/400 + (239*L4^2)/100 - (1690603261718859*cos(t1)^2*cos(t2)^2)/576460752303423488 - ...
    (1690603261718859*cos(t1)^2*cos(t3)^2)/288230376151711744 - (24378*L4*cos(t3)*cos(t4))/25 + ...
    (24378*L4*sin(t3)*sin(t4))/25 + (22466*L3*sin(t4)*sin(t5))/25 + (12189*L3*cos(t3)*sin(t4)*sin(t5))/25 +...
    (12189*L3*cos(t4)*sin(t3)*sin(t5))/25 - (1690603261718859*cos(t1)*cos(t3)*sin(t1)*sin(t3))/288230376151711744 +...
    148084969195448577098115273/115292150460684697600;
M(15)=(1842212*cos(t4))/5 - (9799*L4)/20 + (22503512638915017*cos(t1)^2)/4611686018427387904 +...
    (1690603261718859*cos(t2)^2)/576460752303423488 + (1690603261718859*cos(t3)^2)/576460752303423488 -...
    (239*L3^2*cos(t5)^2)/400 - (44932*L4*cos(t4))/25 + (239*L3^2)/400 + (239*L4^2)/100 -...
    (1690603261718859*cos(t1)^2*cos(t2)^2)/576460752303423488 - (1690603261718859*cos(t1)^2*cos(t3)^2)/288230376151711744 +...
    (22466*L3*sin(t4)*sin(t5))/25 - (1690603261718859*cos(t1)*cos(t3)*sin(t1)*sin(t3))/288230376151711744 +...
    148084969195448577098115273/115292150460684697600;
M(21)=(921106*cos(t4))/5 - (9799*L4)/20 + (30924549306891319*cos(t1)^2)/4611686018427387904 +...
    (1690603261718859*cos(t2)^2)/576460752303423488 + (1690603261718859*cos(t3)^2)/576460752303423488 -...
    (239*L3^2*cos(t5)^2)/400 - (22466*L4*cos(t4))/25 + (239*L3^2)/400 + (239*L4^2)/100 -...
    (1690603261718859*cos(t1)^2*cos(t2)^2)/576460752303423488 - (1690603261718859*cos(t1)^2*cos(t3)^2)/288230376151711744 +...
    (11233*L3*sin(t4)*sin(t5))/25 - (1690603261718859*cos(t1)*cos(t3)*sin(t1)*sin(t3))/288230376151711744 + 231598321612314291030467/4611686018427387904;
M(27)=(1690603261718859*cos(2*t1 + t2 - t3 + t4))/2305843009213693952 - (1690603261718859*cos(t1 + t2 - t3 - t4))/4611686018427387904 +...
    (1690603261718859*cos(2*t1 - t2 + t3 + t4))/9223372036854775808 + (1690603261718859*cos(3*t2 - t1 + t3 + t4))/4611686018427387904 -...
    (1690603261718859*cos(t2 - 2*t1 + 3*t3 + t4))/2305843009213693952 - (1690603261718859*cos(3*t2 - 2*t1 + t3 + t4))/9223372036854775808 +...
    (1690603261718859*cos(2*t1 + 3*t2 + t3 + t4))/9223372036854775808 - (1690603261718859*cos(2*t1 + t2 - t3 - t4))/9223372036854775808 +...
    (1690603261718859*cos(t1 - t2 + t3 + t4))/4611686018427387904 + (10637310166265011*cos(t2 - 2*t1 + t3 + t4))/18446744073709551616 -...
    (10637310166265011*cos(2*t1 + t2 + t3 + t4))/18446744073709551616 - (1690603261718859*cos(t1 + 3*t2 + t3 + t4))/4611686018427387904 -...
    (11233*L3*cos(t4 + t5))/50 - (9799*L3*cos(t5))/80 - (11233*L3*cos(t4 - t5))/50 + (239*L3*L4*cos(t5))/200;
M(33)=(3874897119389575*cos(t5))/4611686018427387904 + (3874897119389575*cos(t1)^2*cos(t5))/4611686018427387904 -...
    (3874897119389575*cos(t1)*cos(t2)*cos(t3)*cos(t4)*sin(t1)*sin(t5))/4611686018427387904 +...
    (3874897119389575*cos(t1)*cos(t2)*sin(t1)*sin(t3)*sin(t4)*sin(t5))/4611686018427387904 +...
    (3874897119389575*cos(t1)*cos(t3)*sin(t1)*sin(t2)*sin(t4)*sin(t5))/4611686018427387904 +...
    (3874897119389575*cos(t1)*cos(t4)*sin(t1)*sin(t2)*sin(t3)*sin(t5))/4611686018427387904;
M(4)=(1690603261718859*cos(t1 - 2*t2))/2305843009213693952 - (1690603261718859*cos(t1 + 2*t2))/2305843009213693952 -...
    (2753519*cos(t2 + t3 + t4))/40 + (4541*L3*cos(t2 + t3 + t4 + t5))/200 - (58077*L3*cos(t2 + t3 + t4 - t5))/400 +...
    (67159*L4*cos(t2 + t3 + t4))/200 - (239*L3^2*cos(t2 + t3 + t4 - 2*t5))/1600 + (239*L3^2*cos(t2 + t3 + t4 + 2*t5))/1600 +...
    (239*L3*L4*cos(t2 + t3 + t4 + t5))/400 + (239*L3*L4*cos(t2 + t3 + t4 - t5))/400;
M(10)=(24162136260015883*cos(2*t1))/9223372036854775808 - (9799*L4)/20 + (1690603261718859*cos(2*t2))/2305843009213693952 +...
    (921106*cos(t4))/5 + (999498*cos(t3)*cos(t4))/5 - (999498*sin(t3)*sin(t4))/5 - (239*L3^2*cos(t5)^2)/400 - (22466*L4*cos(t4))/25 +...
    (239*L3^2)/400 + (239*L4^2)/100 - (1690603261718859*cos(2*t1)*cos(2*t2))/2305843009213693952 -...
    (1690603261718859*cos(2*t1)*cos(t3)^2)/576460752303423488 - (24378*L4*cos(t3)*cos(t4))/25 -...
    (1690603261718859*sin(2*t1)*cos(t3)*sin(t3))/576460752303423488 + (24378*L4*sin(t3)*sin(t4))/25 + (11233*L3*sin(t4)*sin(t5))/25 +...
    (12189*L3*cos(t3)*sin(t4)*sin(t5))/25 + (12189*L3*cos(t4)*sin(t3)*sin(t5))/25 + 463196680911590935827689/9223372036854775808;
M(16)=(921106*cos(t4))/5 - (9799*L4)/20 + (30924549306891319*cos(t1)^2)/4611686018427387904 +...
    (1690603261718859*cos(t2)^2)/576460752303423488 + (1690603261718859*cos(t3)^2)/576460752303423488 -...
    (239*L3^2*cos(t5)^2)/400 - (22466*L4*cos(t4))/25 + (239*L3^2)/400 + (239*L4^2)/100 -...
    (1690603261718859*cos(t1)^2*cos(t2)^2)/576460752303423488 - (1690603261718859*cos(t1)^2*cos(t3)^2)/288230376151711744 +...
    (11233*L3*sin(t4)*sin(t5))/25 - (1690603261718859*cos(t1)*cos(t3)*sin(t1)*sin(t3))/288230376151711744 +...
    231598321612314291030467/4611686018427387904;
M(22)=(10637310166265011*cos(2*t1))/9223372036854775808 - (9799*L4)/20 + (1690603261718859*cos(2*t2))/2305843009213693952 -...
    (239*L3^2*cos(2*t5))/800 + (239*L3^2)/800 + (239*L4^2)/100 - (1690603261718859*cos(2*t1)*cos(2*t2))/2305843009213693952 -...
    (1690603261718859*cos(2*t1)*cos(2*t3))/1152921504606846976 - (1690603261718859*sin(2*t1)*sin(2*t3))/1152921504606846976 +...
    463196680911590935827689/9223372036854775808;
M(28)=(1690603261718859*cos(2*t1 + t2 - t3 + t4))/2305843009213693952 - (1690603261718859*cos(t1 + t2 - t3 - t4))/4611686018427387904 +...
    (1690603261718859*cos(2*t1 - t2 + t3 + t4))/9223372036854775808 + (1690603261718859*cos(3*t2 - t1 + t3 + t4))/4611686018427387904 -...
    (1690603261718859*cos(t2 - 2*t1 + 3*t3 + t4))/2305843009213693952 - (1690603261718859*cos(3*t2 - 2*t1 + t3 + t4))/9223372036854775808 +...
    (1690603261718859*cos(2*t1 + 3*t2 + t3 + t4))/9223372036854775808 - (1690603261718859*cos(2*t1 + t2 - t3 - t4))/9223372036854775808 +...
    (1690603261718859*cos(t1 - t2 + t3 + t4))/4611686018427387904 + (10637310166265011*cos(t2 - 2*t1 + t3 + t4))/18446744073709551616 -...
    (10637310166265011*cos(2*t1 + t2 + t3 + t4))/18446744073709551616 - (1690603261718859*cos(t1 + 3*t2 + t3 + t4))/4611686018427387904 -...
    (9799*L3*cos(t5))/80 + (239*L3*L4*cos(t5))/200;
M(34)=(3874897119389575*cos(t5))/4611686018427387904 + (3874897119389575*cos(t1)^2*cos(t5))/4611686018427387904 -...
    (3874897119389575*cos(t1)*cos(t2)*cos(t3)*cos(t4)*sin(t1)*sin(t5))/4611686018427387904 +...
    (3874897119389575*cos(t1)*cos(t2)*sin(t1)*sin(t3)*sin(t4)*sin(t5))/4611686018427387904 +...
    (3874897119389575*cos(t1)*cos(t3)*sin(t1)*sin(t2)*sin(t4)*sin(t5))/4611686018427387904 +...
    (3874897119389575*cos(t1)*cos(t4)*sin(t1)*sin(t2)*sin(t3)*sin(t5))/4611686018427387904;
M(5)=(1690603261718859*cos(t2 + t3 + t4))/1152921504606846976 -...
    (1690603261718859*cos(t1 + t2 - t3 - t4))/4611686018427387904 +...
    (1690603261718859*cos(3*t2 - t1 + t3 + t4))/4611686018427387904 -...
    (1690603261718859*cos(t3 - t2 + t4))/2305843009213693952 - (1690603261718859*cos(3*t2 + t3 + t4))/2305843009213693952 -...
    (1690603261718859*cos(t1 - t2 + t3 + t4))/4611686018427387904 +...
    (1690603261718859*cos(t1 + 3*t2 + t3 + t4))/4611686018427387904 - (11233*L3*cos(t2 + t3 - t5))/50 +...
    (239*L3^2*cos(t2 + t3 + t4))/400 + (58077*L3*cos(t2 + t3 + t4 + t5))/400 + (12189*L3*cos(t2 + t5))/50 +...
    (4541*L3*cos(t2 + t3 + t4 - t5))/200 - (12189*L3*cos(t2 - t5))/50 + (11233*L3*cos(t2 + t3 + t5))/50 -...
    (239*L3*L4*cos(t2 + t3 + t4 + t5))/400 + (239*L3*L4*cos(t2 + t3 + t4 - t5))/400;
M(11)=(1690603261718859*cos(2*t1 + t2 - t3 + t4))/2305843009213693952 - (1690603261718859*cos(t1 + t2 - t3 - t4))/4611686018427387904 +...
    (1690603261718859*cos(2*t1 - t2 + t3 + t4))/9223372036854775808 + (1690603261718859*cos(3*t2 - t1 + t3 + t4))/4611686018427387904 -...
    (1690603261718859*cos(t2 - 2*t1 + 3*t3 + t4))/2305843009213693952 - (1690603261718859*cos(3*t2 - 2*t1 + t3 + t4))/9223372036854775808 +...
    (1690603261718859*cos(2*t1 + 3*t2 + t3 + t4))/9223372036854775808 - (1690603261718859*cos(2*t1 + t2 - t3 - t4))/9223372036854775808 +...
    (1690603261718859*cos(t1 - t2 + t3 + t4))/4611686018427387904 + (10637310166265011*cos(t2 - 2*t1 + t3 + t4))/18446744073709551616 -...
    (10637310166265011*cos(2*t1 + t2 + t3 + t4))/18446744073709551616 - (1690603261718859*cos(t1 + 3*t2 + t3 + t4))/4611686018427387904 -...
    (12189*L3*cos(t3 + t4 - t5))/50 - (11233*L3*cos(t4 + t5))/50 - (9799*L3*cos(t5))/80 - (11233*L3*cos(t4 - t5))/50 -...
    (12189*L3*cos(t3 + t4 + t5))/50 + (239*L3*L4*cos(t5))/200;
M(17)=(1690603261718859*cos(2*t1 + t2 - t3 + t4))/2305843009213693952 - (1690603261718859*cos(t1 + t2 - t3 - t4))/4611686018427387904 +...
    (1690603261718859*cos(2*t1 - t2 + t3 + t4))/9223372036854775808 + (1690603261718859*cos(3*t2 - t1 + t3 + t4))/4611686018427387904 -...
    (1690603261718859*cos(t2 - 2*t1 + 3*t3 + t4))/2305843009213693952 - (1690603261718859*cos(3*t2 - 2*t1 + t3 + t4))/9223372036854775808 +...
    (1690603261718859*cos(2*t1 + 3*t2 + t3 + t4))/9223372036854775808 - (1690603261718859*cos(2*t1 + t2 - t3 - t4))/9223372036854775808 +...
    (1690603261718859*cos(t1 - t2 + t3 + t4))/4611686018427387904 + (10637310166265011*cos(t2 - 2*t1 + t3 + t4))/18446744073709551616 -...
    (10637310166265011*cos(2*t1 + t2 + t3 + t4))/18446744073709551616 - (1690603261718859*cos(t1 + 3*t2 + t3 + t4))/4611686018427387904 -...
    (11233*L3*cos(t4 + t5))/50 - (9799*L3*cos(t5))/80 - (11233*L3*cos(t4 - t5))/50 + (239*L3*L4*cos(t5))/200;
M(23)=(1690603261718859*cos(2*t1 + t2 - t3 + t4))/2305843009213693952 - (1690603261718859*cos(t1 + t2 - t3 - t4))/4611686018427387904 +...
    (1690603261718859*cos(2*t1 - t2 + t3 + t4))/9223372036854775808 + (1690603261718859*cos(3*t2 - t1 + t3 + t4))/4611686018427387904 -...
    (1690603261718859*cos(t2 - 2*t1 + 3*t3 + t4))/2305843009213693952 - (1690603261718859*cos(3*t2 - 2*t1 + t3 + t4))/9223372036854775808 +...
    (1690603261718859*cos(2*t1 + 3*t2 + t3 + t4))/9223372036854775808 - (1690603261718859*cos(2*t1 + t2 - t3 - t4))/9223372036854775808 +...
    (1690603261718859*cos(t1 - t2 + t3 + t4))/4611686018427387904 + (10637310166265011*cos(t2 - 2*t1 + t3 + t4))/18446744073709551616 -...
    (10637310166265011*cos(2*t1 + t2 + t3 + t4))/18446744073709551616 - (1690603261718859*cos(t1 + 3*t2 + t3 + t4))/4611686018427387904 -...
    (9799*L3*cos(t5))/80 + (239*L3*L4*cos(t5))/200;
M(29)=(239*L3^2)/400 + (10637310166265011*cos(2*t2 - 2*t1 + 2*t3 + 2*t4))/36893488147419103232 +...
    (10637310166265011*cos(2*t1 + 2*t2 + 2*t3 + 2*t4))/36893488147419103232 + (1690603261718859*cos(4*t2 - t1 + 2*t3 + 2*t4))/4611686018427387904 -...
    (1690603261718859*cos(2*t2 - 2*t1 + 4*t3 + 2*t4))/4611686018427387904 - (1690603261718859*cos(4*t2 - 2*t1 + 2*t3 + 2*t4))/18446744073709551616 -...
    (1690603261718859*cos(2*t1 + 4*t2 + 2*t3 + 2*t4))/18446744073709551616 - (10637310166265011*cos(2*t1))/18446744073709551616 -...
    (1690603261718859*cos(2*t2))/4611686018427387904 - (1690603261718859*cos(2*t3 - t1 + 2*t4))/4611686018427387904 -...
    (1690603261718859*cos(2*t1 + 2*t2 + 2*t4))/4611686018427387904 - (1690603261718859*cos(2*t3 - 2*t1 + 2*t4))/18446744073709551616 -...
    (1690603261718859*cos(2*t1 + 2*t3 + 2*t4))/18446744073709551616 - (31911930498795033*cos(2*t2 + 2*t3 + 2*t4))/18446744073709551616 -...
    (5071809785156577*cos(4*t2 + 2*t3 + 2*t4))/9223372036854775808 + (1690603261718859*cos(2*t1 - 2*t2))/9223372036854775808 +...
    (1690603261718859*cos(2*t1 + 2*t2))/9223372036854775808 + (1690603261718859*cos(2*t1 - 2*t3))/2305843009213693952 -...
    (5071809785156577*cos(2*t3 + 2*t4))/9223372036854775808 + (1690603261718859*cos(t1 + 4*t2 + 2*t3 + 2*t4))/4611686018427387904 -...
    (1690603261718859*cos(t1 + 2*t3 + 2*t4))/4611686018427387904 + 58961582686296777/18446744073709551616;
M(35)=(11624691358168725*sin(2*t2)*sin(2*t3)*sin(2*t4)*sin(t5))/18446744073709551616 - (11624691358168725*cos(2*t2)*cos(2*t3)*sin(2*t4)*sin(t5))/18446744073709551616 -...
    (11624691358168725*cos(2*t2)*cos(2*t4)*sin(2*t3)*sin(t5))/18446744073709551616 - (11624691358168725*cos(2*t3)*cos(2*t4)*sin(2*t2)*sin(t5))/18446744073709551616 +...
    (3874897119389575*sin(2*t1)*cos(t2)*cos(t3)*cos(t5)*sin(t4))/9223372036854775808 + (3874897119389575*sin(2*t1)*cos(t2)*cos(t4)*cos(t5)*sin(t3))/9223372036854775808 +...
    (3874897119389575*sin(2*t1)*cos(t3)*cos(t4)*cos(t5)*sin(t2))/9223372036854775808 + (3874897119389575*cos(2*t1)*cos(2*t2)*cos(2*t3)*sin(2*t4)*sin(t5))/18446744073709551616 +...
    (3874897119389575*cos(2*t1)*cos(2*t2)*cos(2*t4)*sin(2*t3)*sin(t5))/18446744073709551616 + (3874897119389575*cos(2*t1)*cos(2*t3)*cos(2*t4)*sin(2*t2)*sin(t5))/18446744073709551616 -...
    (3874897119389575*sin(2*t1)*cos(t5)*sin(t2)*sin(t3)*sin(t4))/9223372036854775808 - (3874897119389575*cos(2*t1)*sin(2*t2)*sin(2*t3)*sin(2*t4)*sin(t5))/18446744073709551616;
M(6)=0;
M(12)=(3874897119389575*cos(t5))/4611686018427387904 + (3874897119389575*cos(t1)^2*cos(t5))/4611686018427387904 -...
    (3874897119389575*cos(t1)*cos(t2)*cos(t3)*cos(t4)*sin(t1)*sin(t5))/4611686018427387904 + (3874897119389575*cos(t1)*cos(t2)*sin(t1)*sin(t3)*sin(t4)*sin(t5))/4611686018427387904 +...
    (3874897119389575*cos(t1)*cos(t3)*sin(t1)*sin(t2)*sin(t4)*sin(t5))/4611686018427387904 + (3874897119389575*cos(t1)*cos(t4)*sin(t1)*sin(t2)*sin(t3)*sin(t5))/4611686018427387904;
M(18)=(3874897119389575*cos(t5))/4611686018427387904 + (3874897119389575*cos(t1)^2*cos(t5))/4611686018427387904 - (3874897119389575*cos(t1)*cos(t2)*cos(t3)*cos(t4)*sin(t1)*sin(t5))/4611686018427387904 +...
    (3874897119389575*cos(t1)*cos(t2)*sin(t1)*sin(t3)*sin(t4)*sin(t5))/4611686018427387904 + (3874897119389575*cos(t1)*cos(t3)*sin(t1)*sin(t2)*sin(t4)*sin(t5))/4611686018427387904 +...
    (3874897119389575*cos(t1)*cos(t4)*sin(t1)*sin(t2)*sin(t3)*sin(t5))/4611686018427387904;
M(24)=(3874897119389575*cos(t5))/4611686018427387904 + (3874897119389575*cos(t1)^2*cos(t5))/4611686018427387904 - (3874897119389575*cos(t1)*cos(t2)*cos(t3)*cos(t4)*sin(t1)*sin(t5))/4611686018427387904 +...
    (3874897119389575*cos(t1)*cos(t2)*sin(t1)*sin(t3)*sin(t4)*sin(t5))/4611686018427387904 + (3874897119389575*cos(t1)*cos(t3)*sin(t1)*sin(t2)*sin(t4)*sin(t5))/4611686018427387904 +...
    (3874897119389575*cos(t1)*cos(t4)*sin(t1)*sin(t2)*sin(t3)*sin(t5))/4611686018427387904;
M(30)=(11624691358168725*sin(2*t2)*sin(2*t3)*sin(2*t4)*sin(t5))/18446744073709551616 - (11624691358168725*cos(2*t2)*cos(2*t3)*sin(2*t4)*sin(t5))/18446744073709551616 -...
    (11624691358168725*cos(2*t2)*cos(2*t4)*sin(2*t3)*sin(t5))/18446744073709551616 - (11624691358168725*cos(2*t3)*cos(2*t4)*sin(2*t2)*sin(t5))/18446744073709551616 +...
    (3874897119389575*sin(2*t1)*cos(t2)*cos(t3)*cos(t5)*sin(t4))/9223372036854775808 + (3874897119389575*sin(2*t1)*cos(t2)*cos(t4)*cos(t5)*sin(t3))/9223372036854775808 +...
    (3874897119389575*sin(2*t1)*cos(t3)*cos(t4)*cos(t5)*sin(t2))/9223372036854775808 + (3874897119389575*cos(2*t1)*cos(2*t2)*cos(2*t3)*sin(2*t4)*sin(t5))/18446744073709551616 +...
    (3874897119389575*cos(2*t1)*cos(2*t2)*cos(2*t4)*sin(2*t3)*sin(t5))/18446744073709551616 + (3874897119389575*cos(2*t1)*cos(2*t3)*cos(2*t4)*sin(2*t2)*sin(t5))/18446744073709551616 -...
    (3874897119389575*sin(2*t1)*cos(t5)*sin(t2)*sin(t3)*sin(t4))/9223372036854775808 - (3874897119389575*cos(2*t1)*sin(2*t2)*sin(2*t3)*sin(2*t4)*sin(t5))/18446744073709551616;
M(36)=((3874897119389575*cos(t1)*cos(t2)*sin(t3)*sin(t4)*sin(t5))/4611686018427387904 - (3874897119389575*cos(t1)*cos(t2)*cos(t3)*cos(t4)*sin(t5))/4611686018427387904 -...
    (3874897119389575*cos(t5)*sin(t1))/4611686018427387904 + (3874897119389575*cos(t1)*cos(t3)*sin(t2)*sin(t4)*sin(t5))/4611686018427387904 +...
    (3874897119389575*cos(t1)*cos(t4)*sin(t2)*sin(t3)*sin(t5))/4611686018427387904)*(cos(t1)*cos(t2)*sin(t3)*sin(t4)*sin(t5) - cos(t1)*cos(t2)*cos(t3)*cos(t4)*sin(t5) -...
    cos(t5)*sin(t1) + cos(t1)*cos(t3)*sin(t2)*sin(t4)*sin(t5) + cos(t1)*cos(t4)*sin(t2)*sin(t3)*sin(t5)) + ((3874897119389575*cos(t1)*cos(t5))/2305843009213693952 -...
    (3874897119389575*cos(t2)*cos(t3)*cos(t4)*sin(t1)*sin(t5))/2305843009213693952 + (3874897119389575*cos(t2)*sin(t1)*sin(t3)*sin(t4)*sin(t5))/2305843009213693952 +...
    (3874897119389575*cos(t3)*sin(t1)*sin(t2)*sin(t4)*sin(t5))/2305843009213693952 + (3874897119389575*cos(t4)*sin(t1)*sin(t2)*sin(t3)*sin(t5))/2305843009213693952)*(cos(t1)*cos(t5) -...
    cos(t2)*cos(t3)*cos(t4)*sin(t1)*sin(t5) + cos(t2)*sin(t1)*sin(t3)*sin(t4)*sin(t5) + cos(t3)*sin(t1)*sin(t2)*sin(t4)*sin(t5) + cos(t4)*sin(t1)*sin(t2)*sin(t3)*sin(t5));

== matlab function PD_trajectory/plant/MATLAB Function4 ==
  data: M input; NumTerm input; Thetadd output
function Thetadd = Response(M,NumTerm)
Thetadd=M\NumTerm;
